simulink model "Robot_Merged_FINAL_for_bilder"  (R2019b)
settings: Solver=VariableStepAuto  StartTime=0.0  StopTime=9.6  RelTol=1e-3  EnableMultiTasking=on
model workspace (MATLAB code in the model file):
  | g=9.81;
  | L1=0.240;
  | L2=0.800;
  | L3=1.050;
  | L4=1.175;
  | L5=0.225;
  | L6=0.200;
  | L7=0.235;
  | L8=0.248;
  | L_BC=0.300;
  | W_BC=0.05;
  | L_BD=0.400;
  | W_BE=W_BC;
values from neighbouring files (symbols this model uses):
  XResults = [p1X p2X p3X]    [PATH_3Dplot.m]    (also in Path_HT.m = [p1X p2X])
undefined symbols (not defined in the file or in its folder): B, Spline, X, Y, Z
libraries: sm_lib x156, nesl_utility x51, simulink x6, robotcorelib x3
(part 5 of 5)

== system Robot_Merged_FINAL_for_bilder/Robot_Controlled/Setup/Subsystem ==
  Torque_In_A : Inport
  Common Gear Constraint : sm_lib/Gears and Couplings/Gears/Common Gear Constraint  GearType=Internal  SpecificationType=CenterDistanceRatio  CenterDistance=100  CenterDistanceUnits=mm  GearRatio=100  BaseGearRadius=10.0  BaseGearRadiusUnits=cm  FollGearRadius=10.0  FollGearRadiusUnits=cm  AssemblyGearRotation=Free
      settings: SourceProductName=Simscape Multibody  SourceProductBaseCode=MS
  Cylindrical Solid3 : sm_lib/Body Elements/Cylindrical Solid  GraphicAmbientColor=[0.15 0.15 0.15 1.0]  BasedOnType=Density  CenterOfMass=[0 0 0]  CenterOfMassUnits=m  GraphicDiffuseColor=[0.5 0.5 0.5]  CylinderLength=0.2  CylinderLengthUnits=m  CylinderRadius=0.05  CylinderRadiusUnits=m  Density=1000  DensityUnits=kg/m^3  DoExposeReferenceFrame=on  GraphicEmissiveColor=[0.0 0.0 0.0 1.0]  ExportEntireGeometry=off  SerializedFrames=<Frames/>  MarkerShape=Sphere  MarkerSize=10  GraphicType=FromGeometry  InertiaType=Custom  Mass=1e-5  MassUnits=kg  MomentsOfInertia=[0 0 0.002]  MomentsOfInertiaUnits=kg*m^2  GraphicOpacity=1.0  ProductsOfInertia=[0 0 0]  ProductsOfInertiaUnits=kg*m^2  GraphicShininess=75  GraphicSpecularColor=[0.5 0.5 0.5 1.0]  GraphicVisPropType=SimpleVisualProperties
  Revolute Joint : sm_lib/Joints/Revolute Joint  JointMode=Normal  SenseConstraintForce=off  SenseConstraintForceX=off  SenseConstraintForceY=off  SenseConstraintForceZ=off  SenseConstraintTorque=off  SenseConstraintTorqueX=off  SenseConstraintTorqueY=off  SenseConstraintTorqueZ=off  SenseTotalForce=off  SenseTotalForceX=off  SenseTotalForceY=off  SenseTotalForceZ=off  SenseTotalTorque=off  SenseTotalTorqueX=off  SenseTotalTorqueY=off  SenseTotalTorqueZ=off  CompositeWrenchDir=FollowerOnBase  CompositeWrenchFrame=BaseFrame  EquilibriumPosition=0  EquilibriumPositionUnits=deg  SpringStiffness=0  SpringStiffnessUnits=N*m/deg  DampingCoefficient=0  DampingCoefficientUnits=N*m/(deg/s)  TorqueActuationMode=InputTorque  MotionActuationMode=ComputedMotion  SensePosition=off  SenseVelocity=off  SenseAcceleration=off  SenseTorqueForce=off  SenseLowerLimitTorqueForce=off  SenseUpperLimitTorqueForce=off  LowerLimitSpecify=off  LowerLimitBound=-90  LowerLimitBoundUnits=deg  LowerLimitStiffness=1e4  LowerLimitStiffnessUnits=N*m/deg  LowerLimitDamping=10  LowerLimitDampingUnits=N*m/(deg/s)  LowerLimitTransitionRegionWidth=0.1  LowerLimitTransitionRegionWidthUnits=deg  UpperLimitSpecify=off  UpperLimitBound=90  UpperLimitBoundUnits=deg  UpperLimitStiffness=1e4  UpperLimitStiffnessUnits=N*m/deg  UpperLimitDamping=10  UpperLimitDampingUnits=N*m/(deg/s)  UpperLimitTransitionRegionWidth=0.1  UpperLimitTransitionRegionWidthUnits=deg  PositionTargetSpecify=off  PositionTargetPriority=High  PositionTargetValue=0  PositionTargetValueUnits=deg  VelocityTargetSpecify=off  VelocityTargetPriority=High  VelocityTargetValue=0  VelocityTargetValueUnits=deg/s
  Rigid Transform : sm_lib/Frames and Transforms/Rigid Transform  TranslationMethod=Cartesian  TranslationStandardOffset=0  TranslationLengthUnit=mm  TranslationStandardAxis=+Z  TranslationCartesianOffset=[100 0 0]  TranslationROffset=0  TranslationROffsetUnits=m  TranslationZOffset=0  TranslationZOffsetUnits=m  TranslationThetaOffset=0  TranslationThetaOffsetUnits=deg  RotationMethod=None  RotationAngleUnits=deg  RotationStandardAxis=+Z  RotationAngle=0.0  RotationArbitraryAxis=[0 0 1]  FollAlignAxisA=+X  BaseAlignAxisA=+Y  FollAlignAxisB=+Y  BaseAlignAxisB=+Z  RotationSequenceAxes=FollowerAxes  RotationSequence=XYX  RotationSequenceAngles=[0 0 0]  RotationSequenceAnglesUnits=deg  RotationMatrix=[1 0 0; 0 1 0; 0 0 1]
  Rigid Transform1 : sm_lib/Frames and Transforms/Rigid Transform  TranslationMethod=Cartesian  TranslationStandardOffset=0  TranslationLengthUnit=m  TranslationStandardAxis=+Z  TranslationCartesianOffset=[0 0 0.01]  TranslationROffset=0  TranslationROffsetUnits=m  TranslationZOffset=0  TranslationZOffsetUnits=m  TranslationThetaOffset=0  TranslationThetaOffsetUnits=deg  RotationMethod=None  RotationAngleUnits=deg  RotationStandardAxis=+Z  RotationAngle=0.0  RotationArbitraryAxis=[0 0 1]  FollAlignAxisA=+X  BaseAlignAxisA=+Y  FollAlignAxisB=+Y  BaseAlignAxisB=+Z  RotationSequenceAxes=FollowerAxes  RotationSequence=XYX  RotationSequenceAngles=[0 0 0]  RotationSequenceAnglesUnits=deg  RotationMatrix=[1 0 0; 0 1 0; 0 0 1]
  Rigid Transform2 : sm_lib/Frames and Transforms/Rigid Transform  TranslationMethod=Cartesian  TranslationStandardOffset=0  TranslationLengthUnit=m  TranslationStandardAxis=+Z  TranslationCartesianOffset=[0 0 0.01]  TranslationROffset=0  TranslationROffsetUnits=m  TranslationZOffset=0  TranslationZOffsetUnits=m  TranslationThetaOffset=0  TranslationThetaOffsetUnits=deg  RotationMethod=None  RotationAngleUnits=deg  RotationStandardAxis=+Z  RotationAngle=0.0  RotationArbitraryAxis=[0 0 1]  FollAlignAxisA=+X  BaseAlignAxisA=+Y  FollAlignAxisB=+Y  BaseAlignAxisB=+Z  RotationSequenceAxes=FollowerAxes  RotationSequence=XYX  RotationSequenceAngles=[0 0 0]  RotationSequenceAnglesUnits=deg  RotationMatrix=[1 0 0; 0 1 0; 0 0 1]
  Simulink-PS Converter : nesl_utility/Simulink-PS Converter  PhysicalDomain=network_engine_domain  SubClassName=ps_input  LeftPortType=input  RightPortType=output  PseudoPeriodic=off  Frequencies=[]  NoiseDistribution=none  NoiseParameters=[]  Unit=1  AffineConversion=off  FilteringAndDerivatives=provide  SimscapeFilterOrder=1  InputFilterTimeConstant=0.001  UdotUserProvided=0
  B_A : PMIOPort  Side=Right
  F_A : PMIOPort  Port=2  Side=Right
  wires:
  Torque_In_A/1 -> Simulink-PS Converter/1
  connections:
  Revolute Joint/RConn1 -- Cylindrical Solid3/RConn1 -- Common Gear Constraint/LConn1
  B_A/RConn1 -- Rigid Transform1/LConn1
  Simulink-PS Converter/RConn1 -- Revolute Joint/LConn2
  Rigid Transform1/RConn1 -- Rigid Transform/LConn1
  Revolute Joint/LConn1 -- Rigid Transform/RConn1
  Rigid Transform2/RConn1 -- Common Gear Constraint/RConn1
  F_A/RConn1 -- Rigid Transform2/LConn1

== matlab function Robot_Merged_FINAL_for_bilder/Robot_HOG/Subsystem/MATLAB Function ==
  settings: updateMethod=DISCRETE  sampleTime=1
  data: x output; y output; P1 input; P2 input; P3 input; P4 input; z output
function [x,y,z] = fcn(P1,P2,P3,P4)

%% Coordinates

T0=0;
T1=1;
T2=2;
T3=3;

%% P1
x1=P1(1);
x1dot=0;
x1dotdot=0;

y1=P1(2);
y1dot=0;
y1dotdot=0;

z1=P1(3);
z1dot=0;
z1dotdot=0;

%% P2
x2=P2(1);
x2dot=0.5;
x2dotdot=0.01;

y2=P2(2);
y2dot=0.01;
y2dotdot=0.010;

z2=P2(3);
z2dot=0.01;
z2dotdot=0.01;

%% P3
x3=P3(1);
x3dot=-0.55;
x3dotdot=0;

y3=P3(2);
y3dot=0.05;
y3dotdot=0;

z3=P3(3);
z3dot=-0.55;
z3dotdot=0;

%% P4
x4=P4(1);
x4dot=0;
x4dotdot=0;

y4=P4(2);
y4dot=0;
y4dotdot=0;

z4=P4(3);
z4dot=0;
z4dotdot=0;


%% Path Generator
t1=[T0:0.001:T1];
t2=[T1:0.001:T2];
t3=[T2:0.001:T3];

Step=0.1;
Counter=1;

X1=[x1
    x1dot
    x1dotdot
    x2
    x2dot];

X2=[x2
    x2dot
    x2dotdot
    x3
    x3dot];

X3=[x3
    x3dot
    x3dotdot
    x4
    x4dot
    x4dotdot];

Y1=[y1
    y1dot
    y1dotdot
    y2
    y2dot];

Y2=[y2
    y2dot
    y2dotdot
    y3
    y3dot];

Y3=[y3
    y3dot
    y3dotdot
    y4
    y4dot
    y4dotdot];


Z1=[z1
    z1dot
    z1dotdot
    z2
    z2dot];
Z2=[z2
    z2dot
    z2dotdot
    z3
    z3dot];
Z3=[z3
    z3dot
    z3dotdot
    z4
    z4dot
    z4dotdot];



F1=[1   T0  T0.^2    T0.^3    T0.^4
    0   1   2*T0     3*T0.^2  4*T0.^3
    0   0   2        6*T0     12*T0.^2
    1   T1  T1.^2    T1.^3    T1.^4
    0   1   2*T1     3*T1.^2  4*T1.^3];

F2=[1   T1  T1.^2    T1.^3    T1.^4    
    0   1   2*T1     3*T1.^2  4*T1.^3  
    0   0   2        6*T1     12*T1.^2 
    1   T2  T2.^2    T2.^3    T2.^4    
    0   1   2*T2     3*T2.^2  4*T2.^3];  


F3=[1   T2  T2.^2    T2.^3    T2.^4    T2.^5
    0   1   2*T2     3*T2.^2  4*T2.^3  5*T2.^4
    0   0   2        6*T2     12*T2.^2 20*T2.^3
    1   T3  T3.^2    T3.^3    T3.^4    T3.^5
    0   1   2*T3     3*T3.^2  4*T3.^3  5*T3.^4
    0   0   2        6*T3     12*T3.^2 20*T3.^3];

CX1=inv(F1)*X1;
CY1=inv(F1)*Y1;
CZ1=inv(F1)*Z1;

CX2=inv(F2)*X2;
CY2=inv(F2)*Y2;
CZ2=inv(F2)*Z2;

CX3=inv(F3)*X3;
CY3=inv(F3)*Y3;
CZ3=inv(F3)*Z3;


p1X=CX1(1)+CX1(2)*t1+CX1(3)*t1.^2+CX1(4)*t1.^3+CX1(5)*t1.^4;
p1Y=CY1(1)+CY1(2)*t1+CY1(3)*t1.^2+CY1(4)*t1.^3+CY1(5)*t1.^4;
p1Z=CZ1(1)+CZ1(2)*t1+CZ1(3)*t1.^2+CZ1(4)*t1.^3+CZ1(5)*t1.^4;

p2X=CX2(1)+CX2(2)*t2+CX2(3)*t2.^2+CX2(4)*t2.^3+CX2(5)*t2.^4;
p2Y=CY2(1)+CY2(2)*t2+CY2(3)*t2.^2+CY2(4)*t2.^3+CY2(5)*t2.^4;
p2Z=CZ2(1)+CZ2(2)*t2+CZ2(3)*t2.^2+CZ2(4)*t2.^3+CZ2(5)*t2.^4;

p3X=CX3(1)+CX3(2)*t3+CX3(3)*t3.^2+CX3(4)*t3.^3+CX3(5)*t3.^4+CX3(6)*t3.^5;
p3Y=CY3(1)+CY3(2)*t3+CY3(3)*t3.^2+CY3(4)*t3.^3+CY3(5)*t3.^4+CY3(6)*t3.^5;
p3Z=CZ3(1)+CZ3(2)*t3+CZ3(3)*t3.^2+CZ3(4)*t3.^3+CZ3(5)*t3.^4+CZ3(6)*t3.^5;

TimeResults=[t1 t2 t3];

XResults=[p1X p2X p3X];
YResults=[p1Y p2Y p3Y];
ZResults=[p1Z p2Z p3Z];

Results=[t1 t2 t3
        p1X p2X p3X
        p1Y p2Y p3Y
        p1Z p2Z p3Z];



x = XResults;

y = YResults;

z = ZResults;
